simulink model "b4_m44_transimpedance"  (R2023a)
settings: Solver=VariableStepAuto  StartTime=0.0  StopTime=0.2  RelTol=1e-3
values from neighbouring files (symbols this model uses):
  w0 = 800    [b4_m45_second_order.m]    (also in b4_m47_third_order_margin.m = 1000)
undefined symbols (not defined in the file or in its folder): A0, Rp, wc
settings Model: Creator=Villou  LastModifiedBy=Villou

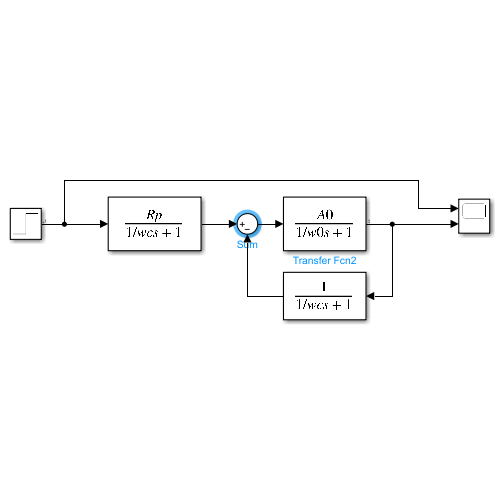
[thumbnail: Simulink's stored preview of the top-level diagram]
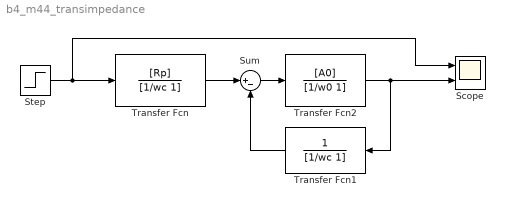
== system b4_m44_transimpedance ==
  Scope : Scope  NumInputPorts=2
  Step : Step  Time=0.01  SampleTime=0
  Sum : Sum  Inputs=|+-
  Transfer Fcn : TransferFcn  Numerator=[Rp]  Denominator=[1/wc 1]
  Transfer Fcn1 : TransferFcn  Denominator=[1/wc 1]
  Transfer Fcn2 : TransferFcn  Numerator=[A0]  Denominator=[1/w0 1]
  wires:
  Transfer Fcn/1 -> Sum/1
  Sum/1 -> Transfer Fcn2/1
  Transfer Fcn1/1 -> Sum/2
  Transfer Fcn2/1 -> Scope/2, Transfer Fcn1/1
  Step/1 -> Scope/1, Transfer Fcn/1
